simulink model "ssrfft_16x4096_noaxis"  (R2019b)
settings: Solver=VariableStepAuto  StartTime=0.0  StopTime=10.0  RelTol=1e-3
libraries: xrbsSSR_Library x14, xbsIndex_r4 x6
settings Model: Creator=jpsmith  LastModifiedBy=one
settings DataIOCC: ReturnWorkspaceOutputs=off
settings DebuggingCC: ArithmeticOperatorsInVariantConditions=warning
settings SFSimCC: CustomCodeUndefinedFunction=UseInterfaceOnly

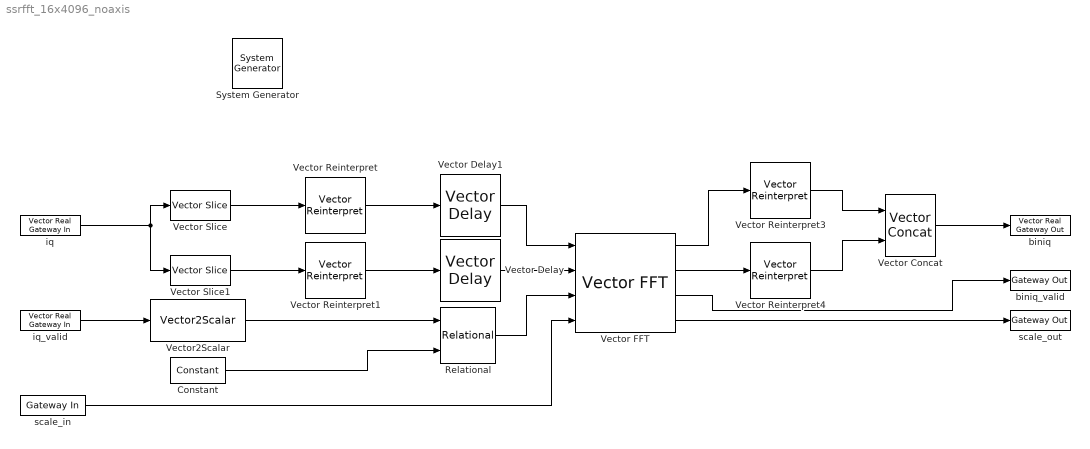
== system ssrfft_16x4096_noaxis ==
  " System Generator" : xbsIndex_r4/ System Generator  Tag=genX  xilinxfamily=zynquplusRFSOC  part=xczu28dr  speed=-2-e  package=ffvg1517  synthesis_tool=Vivado  clock_wrapper=Clock Enables  directory=C:/Users/one/xilinx_projects/ssr_output  proj_type=Vivado  Synth_file=Vivado Synthesis Defaults  Impl_file=Vivado Implementation Defaults  testbench=off  simulink_period=1  sysclk_period=1.81818181  dcm_input_clock_period=10  incr_netlist=off  trim_vbits=Everywhere in SubSystem  dbl_ovrd=According to Block Masks  core_generation=According to Block Masks  run_coregen=off  deprecated_control=off  eval_field=0  block_type=sysgen
  Constant : xbsIndex_r4/Constant  const=65535  gui_display_data_type=Fixed-point  arith_type=Unsigned  n_bits=16  bin_pt=0  preci_type=Single  exp_width=8  frac_width=24  explicit_period=off  period=1  equ=P=C  opselect=C  inp2=PCIN>>17  opr=+  inp1=P  carry=CIN  dbl_ovrd=off  block_type=constant
  Relational : xbsIndex_r4/Relational  mode=a=b  op_type=Bool  en=off  latency=1  dbl_ovrd=off  block_type=relational
  Vector Concat : xrbsSSR_Library/Vector Concat  num_inputs=2  num_inputs_prev=2  sg_ssr=16  sg_ssr_prev=16  dbl_ovrd=off  block_type=concat_ssr  sg_ssr_name=vect_concat
      settings: SourceProductName=Xilinx SSR Blockset  infoedit=The Vector Concat block concatenates two or more inputs of type vector. Output will be cast to an unsigned value with the binary point at zero.
  Vector Delay : xrbsSSR_Library/Vector Delay  sg_latency=1  infoeditControl=Selection of Reset will increase slice count due to use of real FFs and instead of SRLs  en=off  vectorize_en=off  rst=off  reg_retiming=off  block_type=delay_ssr  dbl_ovrd=off  sg_ssr=16  sg_ssr_prev=16  sg_ssr_name=vect_delay
      settings: SourceProductName=Xilinx SSR Blockset
  Vector Delay1 : xrbsSSR_Library/Vector Delay  sg_latency=1  infoeditControl=Selection of Reset will increase slice count due to use of real FFs and instead of SRLs  en=off  vectorize_en=off  rst=off  reg_retiming=off  block_type=delay_ssr  dbl_ovrd=off  sg_ssr=16  sg_ssr_prev=16  sg_ssr_name=vect_delay
      settings: SourceProductName=Xilinx SSR Blockset
  Vector FFT : xrbsSSR_Library/Vector FFT  sg_ssr=16  N=4096  W_high=1  W_low=-17  n_bits=16  bin_pt=15  bram_threshold=258  block_type=fft_ssr
      settings: SourceProductName=Xilinx SSR Blockset
  Vector Reinterpret : xrbsSSR_Library/Vector Reinterpret  sg_ssr=16  sg_ssr_prev=16  force_arith_type=on  arith_type="Signed  (2's comp)"  force_bin_pt=on  bin_pt=15  block_type=reinterpret_ssr
      settings: SourceProductName=Xilinx SSR Blockset  infoedit="The Vector Reinterpret block Changes vector input signal type without altering the binary representation. You can change the signal between signed and unsigned, and relocate the binary point.<br><br>Hardware notes: In hardware this block costs nothing.<br><br>Example:  Suppose the input is 6 bits wide, signed, with 2 fractional bits, and the output is forced to unsigned with 0 fractional bits.  Then an input of -2.0 (1110.00 in binary 2's complement) becomes an output of 56 (111000 in binary)."
  Vector Reinterpret1 : xrbsSSR_Library/Vector Reinterpret  sg_ssr=16  sg_ssr_prev=16  force_arith_type=on  arith_type="Signed  (2's comp)"  force_bin_pt=on  bin_pt=15  block_type=reinterpret_ssr
      settings: SourceProductName=Xilinx SSR Blockset  infoedit="The Vector Reinterpret block Changes vector input signal type without altering the binary representation. You can change the signal between signed and unsigned, and relocate the binary point.<br><br>Hardware notes: In hardware this block costs nothing.<br><br>Example:  Suppose the input is 6 bits wide, signed, with 2 fractional bits, and the output is forced to unsigned with 0 fractional bits.  Then an input of -2.0 (1110.00 in binary 2's complement) becomes an output of 56 (111000 in binary)."
  Vector Reinterpret3 : xrbsSSR_Library/Vector Reinterpret  sg_ssr=16  sg_ssr_prev=16  force_arith_type=on  arith_type=Unsigned  force_bin_pt=on  bin_pt=0  block_type=reinterpret_ssr
      settings: SourceProductName=Xilinx SSR Blockset  infoedit="The Vector Reinterpret block Changes vector input signal type without altering the binary representation. You can change the signal between signed and unsigned, and relocate the binary point.<br><br>Hardware notes: In hardware this block costs nothing.<br><br>Example:  Suppose the input is 6 bits wide, signed, with 2 fractional bits, and the output is forced to unsigned with 0 fractional bits.  Then an input of -2.0 (1110.00 in binary 2's complement) becomes an output of 56 (111000 in binary)."
  Vector Reinterpret4 : xrbsSSR_Library/Vector Reinterpret  sg_ssr=16  sg_ssr_prev=16  force_arith_type=on  arith_type=Unsigned  force_bin_pt=on  bin_pt=0  block_type=reinterpret_ssr
      settings: SourceProductName=Xilinx SSR Blockset  infoedit="The Vector Reinterpret block Changes vector input signal type without altering the binary representation. You can change the signal between signed and unsigned, and relocate the binary point.<br><br>Hardware notes: In hardware this block costs nothing.<br><br>Example:  Suppose the input is 6 bits wide, signed, with 2 fractional bits, and the output is forced to unsigned with 0 fractional bits.  Then an input of -2.0 (1110.00 in binary 2's complement) becomes an output of 56 (111000 in binary)."
  Vector Slice : xrbsSSR_Library/Vector Slice  nbits=16  sg_ssr=16  sg_ssr_prev=16  boolean_output=off  mode=Lower Bit Location + Width  bit1=0  base1=LSB of Input  bit0=16  base0=LSB of Input  dbl_ovrd=off  block_type=slice_ssr  sg_ssr_name=vect_slice
      settings: SourceProductName=Xilinx SSR Blockset  infoedit="The Vector Slice block supports input of vector types. Extracts a given range of bits from each sample of input vector and presents it at the output.  The output type is ordinarily unsigned with binary point at zero, but can be Boolean when the slice is one bit wide.<br><br>Hardware notes: In hardware this block costs nothing."
  Vector Slice1 : xrbsSSR_Library/Vector Slice  nbits=16  sg_ssr=16  sg_ssr_prev=16  boolean_output=off  mode=Lower Bit Location + Width  bit1=32  base1=LSB of Input  bit0=0  base0=LSB of Input  dbl_ovrd=off  block_type=slice_ssr  sg_ssr_name=vect_slice
      settings: SourceProductName=Xilinx SSR Blockset  infoedit="The Vector Slice block supports input of vector types. Extracts a given range of bits from each sample of input vector and presents it at the output.  The output type is ordinarily unsigned with binary point at zero, but can be Boolean when the slice is one bit wide.<br><br>Hardware notes: In hardware this block costs nothing."
  Vector2Scalar : xrbsSSR_Library/Vector2Scalar  sg_ssr=16  sg_ssr_prev=16  sg_ssr_name=vect_Vector2Scalar  block_type=vector2scalar_ssr
      settings: SourceProductName=Xilinx SSR Blockset
  biniq : xrbsSSR_Library/Vector Real Gateway Out  inherit_from_input=off  hdl_port=on  rows=1  columns=1  UseAsDAC=off  DACChannel='1'  interface=None  automatic_assignment=on  address_offset=hex2dec('00')  intf_name=''  intf_description=''  timing_constraint=None  locs_specified=off  LOCs={}  io_standard={}  block_type=realgatewayout_ssr  sg_ssr=16  sg_ssr_prev=16  sg_ssr_name=vect_real_gwayout  name_prev=biniq
      settings: SourceProductName=Xilinx SSR Blockset  infoedit=The Vector Real Gateway out block converts Xilinx fixed-point or floating-point type vector inputs into vector ouputs of type Simulink integer, single, double, or fixed-point.<br><br>Hardware notes: In hardware these blocks become top level output ports or are discarded, depending on how they are configured.
  "biniq_valid " : xbsIndex_r4/Gateway Out  inherit_from_input=off  hdl_port=on  rows=1  columns=1  UseAsDAC=off  DACChannel='1'  interface=None  automatic_assignment=on  address_offset=hex2dec('00')  intf_name=''  intf_description=''  timing_constraint=None  locs_specified=off  LOCs={}  io_standard={}  block_type=gatewayout
  iq : xrbsSSR_Library/Vector Real Gateway In  gui_display_data_type=Fixed-point  arith_type=Unsigned  n_bits=32  bin_pt=0  preci_type=Single  exp_width=8  frac_width=24  quantization="Round  (unbiased: +/- Inf)"  overflow=Saturate  period=1  sg_ssr=16  sg_ssr_prev=16  UseAsADC=off  ADCChannel='1'  interface=None  interface_prev=1  automatic_assignment=off  address_offset=hex2dec('00')  intf_name=''  intf_description=''  default_value=0  timing_constraint=None  locs_specified=off  LOCs={}  io_standard={}  hdl_port=on  dbl_ovrd=off  block_type=realgatewayin_ssr  name_prev=iq
      settings: SourceProductName=Xilinx SSR Blockset  infoedit=The Vector Real Gateway in block converts Vector inputs of type Simulink integer, single, double and fixed-point to Xilinx fixed-point or floating-point data type.<br><br>Hardware notes: In hardware these blocks become top level input ports.
  iq_valid : xrbsSSR_Library/Vector Real Gateway In  gui_display_data_type=Boolean  arith_type=Boolean  n_bits=16  bin_pt=14  preci_type=Single  exp_width=8  frac_width=24  quantization="Round  (unbiased: +/- Inf)"  overflow=Saturate  period=1  sg_ssr=16  sg_ssr_prev=16  UseAsADC=off  ADCChannel='1'  interface=None  interface_prev=1  automatic_assignment=off  address_offset=hex2dec('00')  intf_name=''  intf_description=''  default_value=0  timing_constraint=None  locs_specified=off  LOCs={}  io_standard={}  hdl_port=on  dbl_ovrd=off  block_type=realgatewayin_ssr  name_prev=iq_valid
      settings: SourceProductName=Xilinx SSR Blockset  infoedit=The Vector Real Gateway in block converts Vector inputs of type Simulink integer, single, double and fixed-point to Xilinx fixed-point or floating-point data type.<br><br>Hardware notes: In hardware these blocks become top level input ports.
  scale_in : xbsIndex_r4/Gateway In  gui_display_data_type=Fixed-point  arith_type=Unsigned  n_bits=12  bin_pt=0  preci_type=Single  exp_width=8  frac_width=24  rows=1  columns=1  quantization="Round  (unbiased: +/- Inf)"  overflow=Saturate  period=1  UseAsADC=off  ADCChannel='1'  interface=None  automatic_assignment=on  address_offset=hex2dec('00')  intf_name=''  intf_description=''  default_value=0  timing_constraint=None  locs_specified=off  LOCs={}  io_standard={}  inherit_from_input=off  hdl_port=on  dbl_ovrd=off  block_type=gatewayin
  scale_out : xbsIndex_r4/Gateway Out  inherit_from_input=off  hdl_port=on  rows=1  columns=1  UseAsDAC=off  DACChannel='1'  interface=None  automatic_assignment=on  address_offset=hex2dec('00')  intf_name=''  intf_description=''  timing_constraint=None  locs_specified=off  LOCs={}  io_standard={}  block_type=gatewayout
  wires:
  iq/1 -> Vector Slice/1, Vector Slice1/1
  Vector FFT/1 -> Vector Reinterpret3/1
  Vector FFT/2 -> Vector Reinterpret4/1
  Vector Slice/1 -> Vector Reinterpret/1
  Vector Reinterpret/1 -> Vector Delay1/1
  Vector Slice1/1 -> Vector Reinterpret1/1
  Vector Reinterpret1/1 -> Vector Delay/1
  scale_in/1 -> Vector FFT/4
  Vector FFT/3 -> "biniq_valid "/1
  Vector FFT/4 -> scale_out/1
  Vector Reinterpret4/1 -> Vector Concat/2
  Vector Reinterpret3/1 -> Vector Concat/1
  Vector Concat/1 -> biniq/1
  iq_valid/1 -> Vector2Scalar/1
  Vector2Scalar/1 -> Relational/1
  Constant/1 -> Relational/2
  Relational/1 -> Vector FFT/3
  Vector Delay1/1 -> Vector FFT/1
  Vector Delay/1 -> Vector FFT/2
